simulink model "MagLev_Nonlinear_vs_Linear"  (R2019b)
settings: Solver=VariableStepAuto  StartTime=0.0  StopTime=15.0  RelTol=1e-3
libraries: cstblocks x3, simulink x2
settings Model: Creator=Santoshi Kulkarni  LastModifiedBy=Santoshi Kulkarni

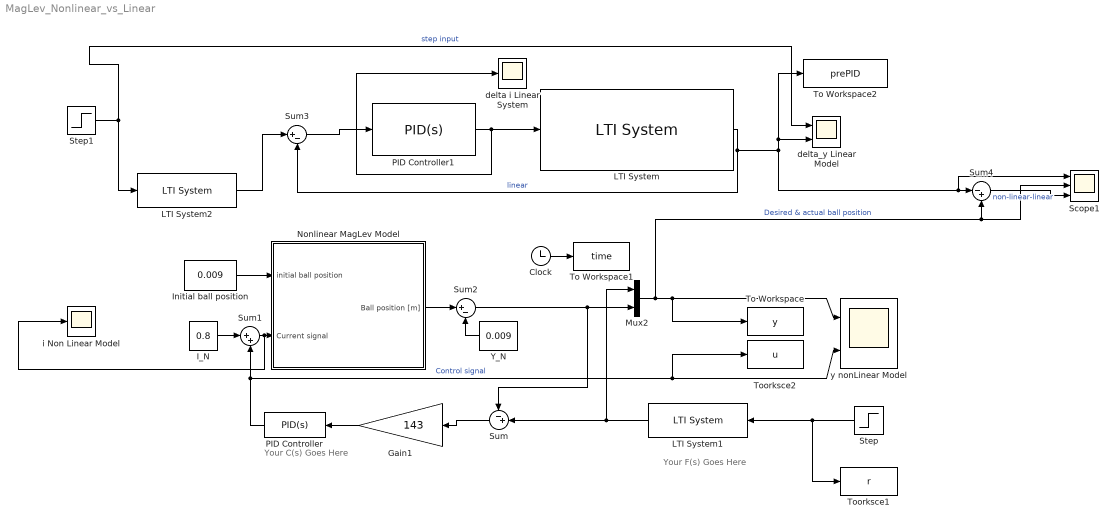
== system MagLev_Nonlinear_vs_Linear ==
  note: Your F(s) Goes Here
  note: Your C(s) Goes Here
  " i Non Linear Model" : Scope
  " y nonLinear Model" : Scope  NumInputPorts=2
  Clock : Clock
  Gain1 : Gain  Gain=143
  I_N : Constant  Value=0.8
  Initial ball position : Constant  Value=0.009
  LTI System : cstblocks/LTI System  sys=tf(-3458,[1 0 -2178])  IC=[]
  LTI System1 : cstblocks/LTI System  sys=tf(5,[1 5])  IC=[]
  LTI System2 : cstblocks/LTI System  sys=tf(5,[1 5])  IC=[]
  Mux2 : Mux  Inputs=2
  Nonlinear MagLev Model : Subsystem
  PID Controller : simulink/Continuous/PID Controller  Controller=PID  Form=Parallel  TimeDomain=Continuous-time  SampleTime=-1  IntegratorMethod=Forward Euler  FilterMethod=Forward Euler  ControllerParametersSource=internal  P=-4.45  I=-3.09  D=-0.0532  UseFilter=on  N=100  TunerSelectOption=Transfer Function Based (PID Tuner App)  InitialConditionSource=internal  InitialConditionForIntegrator=0  InitialConditionForFilter=0  DifferentiatorICPrevScaledInput=0  ExternalReset=none  TrackingMode=off  Kt=1  LimitOutput=off  UpperSaturationLimit=inf  LowerSaturationLimit=-inf  LinearizeAsGain=on  AntiWindupMode=none  Kb=1  POutMin=[]  POutMax=[]  IOutMin=[]  IOutMax=[]  DOutMin=[]  DOutMax=[]  NOutMin=[]  NOutMax=[]  SumOutMin=[]  SumOutMax=[]  SaturationOutMin=[]  SaturationOutMax=[]  PParamMin=[]  PParamMax=[]  IParamMin=[]  IParamMax=[]  DParamMin=[]  DParamMax=[]  NParamMin=[]  NParamMax=[]  KbParamMin=[]  KbParamMax=[]  KtParamMin=[]  KtParamMax=[]  KbOutMin=[]  KbOutMax=[]  KtOutMin=[]  KtOutMax=[]  IntegratorOutMin=[]  IntegratorOutMax=[]  FilterOutMin=[]  FilterOutMax=[]  SumI1OutMin=[]  SumI1OutMax=[]  SumI2OutMin=[]  SumI2OutMax=[]  SumI3OutMin=[]  SumI3OutMax=[]  SumI4OutMin=[]  SumI4OutMax=[]  SumDOutMin=[]  SumDOutMax=[]  DifferentiatorOutMin=[]  DifferentiatorOutMax=[]  FilterDiffOutCoefMin=[]  FilterDiffOutCoefMax=[]  ReciprocalOutMin=[]  ReciprocalOutMax=[]  SumDenOutMin=[]  SumDenOutMax=[]  SumNumOutMin=[]  SumNumOutMax=[]  DivideOutMin=[]  DivideOutMax=[]  IntegratorContinuousStateAttributes=''  IntegratorStateMustResolveToSignalObject=off  IntegratorRTWStateStorageClass=Auto  FilterContinuousStateAttributes=''  FilterStateMustResolveToSignalObject=off  FilterRTWStateStorageClass=Auto  ParallelPVariant=InternalParameters  IdealPVariant=Disabled  IVariant=InternalParameters  DVariant=InternalParameters  IntegratorVariant=Continuous  SatVariant=Disabled  AWVariant=Passthrough  PCopyVariant=Disabled  TRVariant=Disabled  FdbkBlocksVariant=Forward  IdealPFdbkVariant=Disabled  SatFdbkVariant=Disabled  DerivativeFilterVariant=ContFilter  NVariant=InternalParameters  NCopyVariant=Disabled  FilterICVariant=InternalICsFilter  IntegratorICVariant=InternalICs  ExternalResetVariant=Disabled  TRSumVariant=Passthrough  SumFdbkVariant=Disabled  SumVariant=Sum_PID
  PID Controller1 : simulink/Continuous/PID Controller  Controller=PID  Form=Parallel  TimeDomain=Continuous-time  SampleTime=-1  IntegratorMethod=Forward Euler  FilterMethod=Forward Euler  ControllerParametersSource=internal  P=-4.45  I=-3.09  D=-0.0532  UseFilter=on  N=100  TunerSelectOption=Transfer Function Based (PID Tuner App)  InitialConditionSource=internal  InitialConditionForIntegrator=0  InitialConditionForFilter=0  DifferentiatorICPrevScaledInput=0  ExternalReset=none  TrackingMode=off  Kt=1  LimitOutput=off  UpperSaturationLimit=inf  LowerSaturationLimit=-inf  LinearizeAsGain=on  AntiWindupMode=none  Kb=1  POutMin=[]  POutMax=[]  IOutMin=[]  IOutMax=[]  DOutMin=[]  DOutMax=[]  NOutMin=[]  NOutMax=[]  SumOutMin=[]  SumOutMax=[]  SaturationOutMin=[]  SaturationOutMax=[]  PParamMin=[]  PParamMax=[]  IParamMin=[]  IParamMax=[]  DParamMin=[]  DParamMax=[]  NParamMin=[]  NParamMax=[]  KbParamMin=[]  KbParamMax=[]  KtParamMin=[]  KtParamMax=[]  KbOutMin=[]  KbOutMax=[]  KtOutMin=[]  KtOutMax=[]  IntegratorOutMin=[]  IntegratorOutMax=[]  FilterOutMin=[]  FilterOutMax=[]  SumI1OutMin=[]  SumI1OutMax=[]  SumI2OutMin=[]  SumI2OutMax=[]  SumI3OutMin=[]  SumI3OutMax=[]  SumI4OutMin=[]  SumI4OutMax=[]  SumDOutMin=[]  SumDOutMax=[]  DifferentiatorOutMin=[]  DifferentiatorOutMax=[]  FilterDiffOutCoefMin=[]  FilterDiffOutCoefMax=[]  ReciprocalOutMin=[]  ReciprocalOutMax=[]  SumDenOutMin=[]  SumDenOutMax=[]  SumNumOutMin=[]  SumNumOutMax=[]  DivideOutMin=[]  DivideOutMax=[]  IntegratorContinuousStateAttributes=''  IntegratorStateMustResolveToSignalObject=off  IntegratorRTWStateStorageClass=Auto  FilterContinuousStateAttributes=''  FilterStateMustResolveToSignalObject=off  FilterRTWStateStorageClass=Auto  ParallelPVariant=InternalParameters  IdealPVariant=Disabled  IVariant=InternalParameters  DVariant=InternalParameters  IntegratorVariant=Continuous  SatVariant=Disabled  AWVariant=Passthrough  PCopyVariant=Disabled  TRVariant=Disabled  FdbkBlocksVariant=Forward  IdealPFdbkVariant=Disabled  SatFdbkVariant=Disabled  DerivativeFilterVariant=ContFilter  NVariant=InternalParameters  NCopyVariant=Disabled  FilterICVariant=InternalICsFilter  IntegratorICVariant=InternalICs  ExternalResetVariant=Disabled  TRSumVariant=Passthrough  SumFdbkVariant=Disabled  SumVariant=Sum_PID
  Scope1 : Scope  NumInputPorts=3
  Step : Step  Time=0  After=0.002  SampleTime=0
  Step1 : Step  Time=0  After=0.002  SampleTime=0
  Sum : Sum  Inputs=-+|
  Sum1 : Sum  Inputs=|++
  Sum2 : Sum  Inputs=|+-
  Sum3 : Sum  Inputs=|+-
  Sum4 : Sum  Inputs=|-+
  To Workspace : ToWorkspace  VariableName=y  SampleTime=0.01
  To Workspace1 : ToWorkspace  VariableName=time  SampleTime=0.01
  To Workspace2 : ToWorkspace  VariableName=prePID  SampleTime=-1
  Toorksce1 : ToWorkspace  VariableName=r  SampleTime=0.01
  Toorksce2 : ToWorkspace  VariableName=u  SampleTime=0.01
  Y_N : Constant  Value=0.009
  delta i Linear System : Scope
  delta_y Linear Model : Scope  NumInputPorts=2
  wires:
  Initial ball position/1 -> Nonlinear MagLev Model/1(initial ball position)
  Gain1/1 -> PID Controller/1
  Y_N/1 -> Sum2/2
  Step1/1 -> delta_y Linear Model/1, LTI System2/1  "step input"
  Clock/1 -> To Workspace1/1
  Sum2/1 -> Mux2/2, Sum/1
  Sum3/1 -> PID Controller1/1
  PID Controller/1 -> " y nonLinear Model"/2, Toorksce2/1, Sum1/2  "Control signal"
  Nonlinear MagLev Model/1(Ball position [m]) -> Sum2/1
  Sum/1 -> Gain1/1
  Sum4/1 -> Scope1/3  "non-linear-linear"
  Step/1 -> LTI System1/1, Toorksce1/1
  LTI System/1 -> Sum3/2, Scope1/1, Sum4/1, To Workspace2/1, delta_y Linear Model/2  "linear"
  Sum1/1 -> " i Non Linear Model"/1, Nonlinear MagLev Model/2(Current signal)
  Mux2/1 -> " y nonLinear Model"/1, To Workspace/1, Scope1/2, Sum4/2  "Desired & actual ball position"
  PID Controller1/1 -> delta i Linear System/1, LTI System/1
  I_N/1 -> Sum1/1
  LTI System2/1 -> Sum3/1
  LTI System1/1 -> Mux2/1, Sum/2

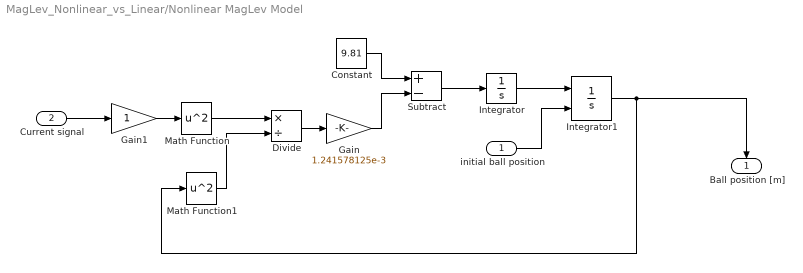
== system MagLev_Nonlinear_vs_Linear/Nonlinear MagLev Model ==
  initial ball position : Inport
  Current signal : Inport  Port=2
  Constant : Constant  Value=9.81
  Divide : Product  Inputs=*/
  Gain : Gain  Gain=1.241578125e-3
  Gain1 : Gain
  Integrator : Integrator
  Integrator1 : Integrator  InitialConditionSource=external
  Math Function : Math  Operator=square  SaturateOnIntegerOverflow=on
  Math Function1 : Math  Operator=square  SaturateOnIntegerOverflow=on
  Subtract : Sum  Inputs=+-
  Ball position [m] : Outport
  wires:
  Gain1/1 -> Math Function/1
  Current signal/1 -> Gain1/1
  initial ball position/1 -> Integrator1/2
  Integrator1/1 -> Math Function1/1, Ball position [m]/1
  Integrator/1 -> Integrator1/1
  Subtract/1 -> Integrator/1
  Gain/1 -> Subtract/2
  Divide/1 -> Gain/1
  Math Function1/1 -> Divide/2
  Math Function/1 -> Divide/1
  Constant/1 -> Subtract/1
